simulink model "rlMobileRobotMdl"  (R2020a)
settings: Solver=FixedStepAuto  StartTime=0.0  StopTime=15  FixedStep=0.01  RelTol=1e-3
model workspace (MAT data in the model file):
  Dl = 0.09
  Dr = 0.09
  Kl = 1
  Kr = 1
  L = 0.45
  Sig = Simulink.Signal
  Sig.DataType = 'auto'
  Sig.Dimensions = -1
  Sig.DimensionsMode = 'auto'
  Sig.Complexity = 'auto'
  Sig.SampleTime = -1
  Sig.SamplingMode = 'auto'
  Tl = 0.05
  Tr = 0.05
  theta0 = 2.3562
  x0 = 0.3536
  y0 = 0.3536
libraries: cstblocks x2, rllib x1, simulink x1
settings Model: OrderedModelArguments=off  Creator=Student  LastModifiedBy=Student

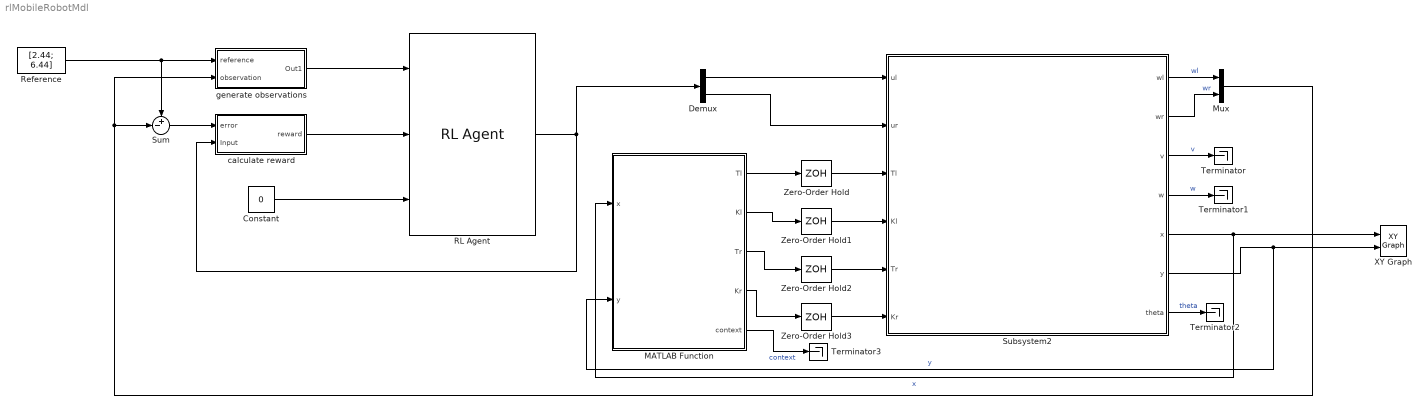
== system rlMobileRobotMdl ==
  Constant : Constant  Value=0
  Demux : Demux  Outputs=2
  MATLAB Function : MATLAB Function  TreatAsAtomicUnit=on
  Mux : Mux  Inputs=2
  RL Agent : rllib/RL Agent  Agent=agent  ProvideReward=on  ProvideIsDone=on  ProvideCumRwd=off  TreatAsDirectFeedthrough=on  CollectLoggedSignals=on  CollectModelStates=on
  Reference : Constant  Value=[2.44; 6.44]
  Subsystem2 : Subsystem
  Sum : Sum  Inputs=+-|
  Terminator{,1..3} (4 alike) : Terminator
  XY Graph : simulink/Sinks/XY Graph  xmin=-1  xmax=1  ymin=-1  ymax=1  st=-1
  Zero-Order Hold{,1..3} (4 alike) : ZeroOrderHold  SampleTime=-1
  calculate reward : Subsystem
  generate observations : Subsystem
  wires:
  calculate reward/1(reward) -> RL Agent/2
  RL Agent/1 -> calculate reward/2("Input "), Demux/1
  Constant/1 -> RL Agent/3
  generate observations/1(Out1) -> RL Agent/1
  Demux/1 -> Subsystem2/1(ul)
  Demux/2 -> Subsystem2/2(ur)
  Reference/1 -> Sum/1, generate observations/1(reference)
  Subsystem2/1(wl) -> Mux/1  "wl"
  Subsystem2/2(wr) -> Mux/2  "wr"
  Mux/1 -> generate observations/2(observation), Sum/2
  Sum/1 -> calculate reward/1(error)
  Subsystem2/5(x) -> MATLAB Function/1(x), XY Graph/1  "x"
  Subsystem2/6(y) -> MATLAB Function/2(y), XY Graph/2  "y"
  Subsystem2/3(v) -> Terminator/1  "v"
  Subsystem2/4(w) -> Terminator1/1  "w"
  Subsystem2/7(theta) -> Terminator2/1  "theta"
  MATLAB Function/1(Tl) -> Zero-Order Hold/1
  Zero-Order Hold/1 -> Subsystem2/3(Tl)
  MATLAB Function/2(Kl) -> Zero-Order Hold1/1
  Zero-Order Hold1/1 -> Subsystem2/4(Kl)
  Zero-Order Hold2/1 -> Subsystem2/5(Tr)
  MATLAB Function/3(Tr) -> Zero-Order Hold2/1
  MATLAB Function/4(Kr) -> Zero-Order Hold3/1
  Zero-Order Hold3/1 -> Subsystem2/6(Kr)
  MATLAB Function/5(context) -> Terminator3/1  "context"

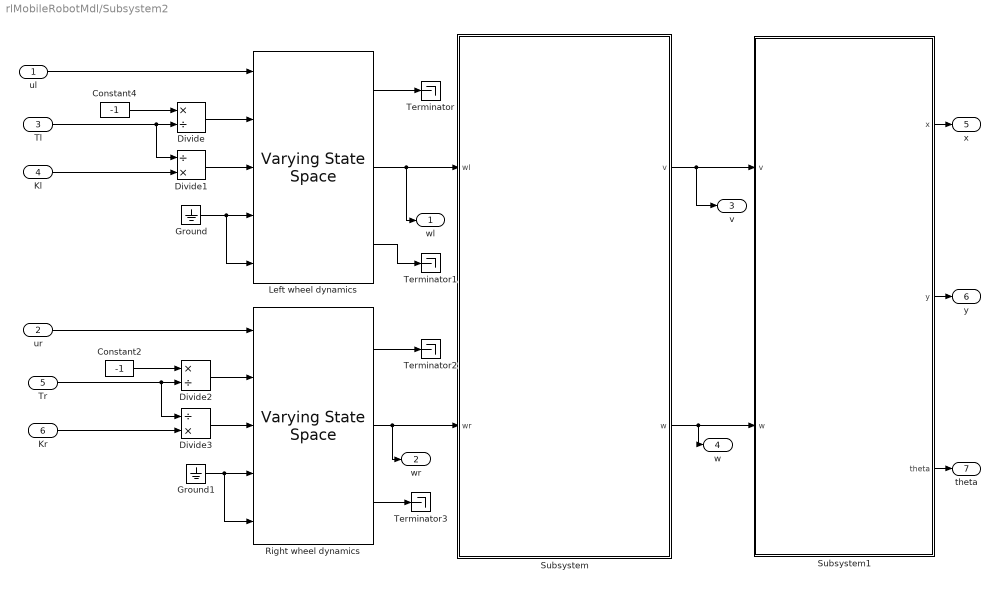
== system rlMobileRobotMdl/Subsystem2 ==
  ul : Inport
  ur : Inport  Port=2
  Tl : Inport  Port=3
  Kl : Inport  Port=4
  Tr : Inport  Port=5
  Kr : Inport  Port=6
  Constant2 : Constant  Value=-1
  Constant4 : Constant  Value=-1
  Divide : Product  Inputs=*/
  Divide1 : Product  Inputs=/*
  Divide2 : Product  Inputs=*/
  Divide3 : Product  Inputs=/*
  Ground : Ground
  Ground1 : Ground
  Left wheel dynamics : cstblocks/Linear Parameter Varying/Varying State Space  x0=0  xNames=''  OutputX=on  OutputDX=on
  Right wheel dynamics : cstblocks/Linear Parameter Varying/Varying State Space  x0=0  xNames=''  OutputX=on  OutputDX=on
  Subsystem : Subsystem
  Subsystem1 : Subsystem
  Terminator{,1..3} (4 alike) : Terminator
  wl : Outport
  wr : Outport  Port=2
  v : Outport  Port=3
  w : Outport  Port=4
  x : Outport  Port=5
  y : Outport  Port=6
  theta : Outport  Port=7
  wires:
  Right wheel dynamics/2 -> wr/1, Subsystem/2(wr)
  Divide/1 -> Left wheel dynamics/2
  Subsystem1/2(y) -> y/1
  Subsystem/1(v) -> v/1, Subsystem1/1(v)
  Left wheel dynamics/2 -> wl/1, Subsystem/1(wl)
  Subsystem/2(w) -> w/1, Subsystem1/2(w)
  ul/1 -> Left wheel dynamics/1
  ur/1 -> Right wheel dynamics/1
  Subsystem1/3(theta) -> theta/1
  Subsystem1/1(x) -> x/1
  Constant4/1 -> Divide/1
  Tl/1 -> Divide1/1, Divide/2
  Divide1/1 -> Left wheel dynamics/3
  Kl/1 -> Divide1/2
  Ground/1 -> Left wheel dynamics/5, Left wheel dynamics/4
  Tr/1 -> Divide3/1, Divide2/2
  Divide3/1 -> Right wheel dynamics/3
  Divide2/1 -> Right wheel dynamics/2
  Constant2/1 -> Divide2/1
  Kr/1 -> Divide3/2
  Ground1/1 -> Right wheel dynamics/5, Right wheel dynamics/4
  Left wheel dynamics/1 -> Terminator/1
  Left wheel dynamics/3 -> Terminator1/1
  Right wheel dynamics/1 -> Terminator2/1
  Right wheel dynamics/3 -> Terminator3/1

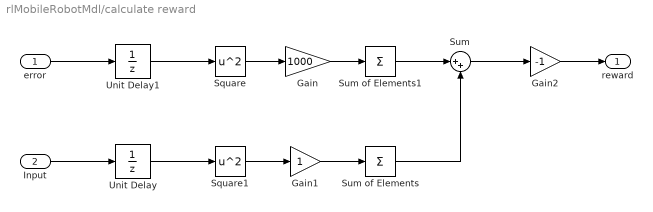
== system rlMobileRobotMdl/calculate reward ==
  error : Inport
  "Input " : Inport  Port=2
  Gain : Gain  Gain=1000
  Gain1 : Gain
  Gain2 : Gain  Gain=-1
  Square : Math  Operator=square  SaturateOnIntegerOverflow=on
  Square1 : Math  Operator=square  SaturateOnIntegerOverflow=on
  Sum : Sum  Inputs=|++
  Sum of Elements : Sum  Inputs=+
  Sum of Elements1 : Sum  Inputs=+
  Unit Delay : UnitDelay  SampleTime=-1  HasFrameUpgradeWarning=on
  Unit Delay1 : UnitDelay  InitialCondition=1  SampleTime=-1  HasFrameUpgradeWarning=on
  reward : Outport
  wires:
  Square/1 -> Gain/1
  Sum/1 -> Gain2/1
  Gain2/1 -> reward/1
  "Input "/1 -> Unit Delay/1
  Unit Delay/1 -> Square1/1
  Square1/1 -> Gain1/1
  error/1 -> Unit Delay1/1
  Unit Delay1/1 -> Square/1
  Gain1/1 -> Sum of Elements/1
  Gain/1 -> Sum of Elements1/1
  Sum of Elements/1 -> Sum/2
  Sum of Elements1/1 -> Sum/1

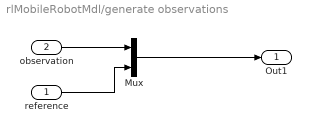
== system rlMobileRobotMdl/generate observations ==
  reference : Inport
  observation : Inport  Port=2
  Mux : Mux  Inputs=2
  Out1 : Outport
  wires:
  observation/1 -> Mux/1
  reference/1 -> Mux/2
  Mux/1 -> Out1/1

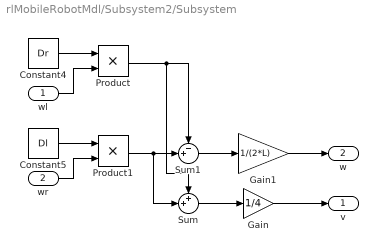
== system rlMobileRobotMdl/Subsystem2/Subsystem ==
  wl : Inport
  wr : Inport  Port=2
  Constant4 : Constant  Value=Dr
  Constant5 : Constant  Value=Dl
  Gain : Gain  Gain=1/4
  Gain1 : Gain  Gain=1/(2*L)
  Product : Product
  Product1 : Product
  Sum : Sum  Inputs=++|
  Sum1 : Sum  Inputs=-+|
  v : Outport
  w : Outport  Port=2
  wires:
  Product1/1 -> Sum1/2, Sum/2
  Gain1/1 -> w/1
  Sum1/1 -> Gain1/1
  Sum/1 -> Gain/1
  Gain/1 -> v/1
  wr/1 -> Product1/2
  wl/1 -> Product/2
  Constant4/1 -> Product/1
  Constant5/1 -> Product1/1
  Product/1 -> Sum1/1, Sum/1

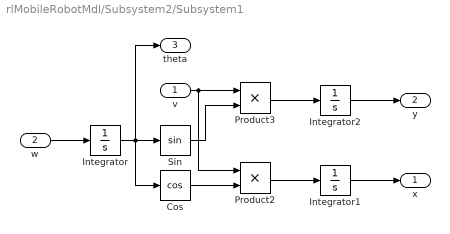
== system rlMobileRobotMdl/Subsystem2/Subsystem1 ==
  v : Inport
  w : Inport  Port=2
  Cos : Trigonometry  Operator=cos
  Integrator : Integrator  InitialCondition=theta0
  Integrator1 : Integrator  InitialCondition=x0
  Integrator2 : Integrator  InitialCondition=y0
  Product2 : Product
  Product3 : Product
  Sin : Trigonometry
  x : Outport
  y : Outport  Port=2
  theta : Outport  Port=3
  wires:
  Integrator/1 -> Sin/1, theta/1, Cos/1
  Sin/1 -> Product3/2
  Cos/1 -> Product2/2
  w/1 -> Integrator/1
  v/1 -> Product3/1, Product2/1
  Product2/1 -> Integrator1/1
  Integrator1/1 -> x/1
  Product3/1 -> Integrator2/1
  Integrator2/1 -> y/1

== matlab function rlMobileRobotMdl/MATLAB Function ==
  data: x input; Tl output; y input; Kl output; Tr output; Kr output; context output
function [Tl, Kl, Tr, Kr, context] = fcn(x, y)
    if (x >= 0 && y >= 0) 
        Tl = 0.05;  Kl = 1;    Tr = 0.05;  Kr = 1;    context = 1;
    elseif (x <  0 && y >= 0)
        Tl = 0.05;  Kl = 1;    Tr = 0.055; Kr = 0.95; context = 2;
    elseif (x < 0 && y <  0)
        Tl = 0.055; Kl = 0.95; Tr = 0.055; Kr = 0.95; context = 3;
else
        Tl = 0.055; Kl = 0.95; Tr = 0.05; Kr = 1;    context = 4;
    end
end
